simulink model "MPC_backend_adaptive"  (R2026a)
settings: Solver=VariableStepAuto
model workspace (MAT data in the model file):
  kappa_ref = 1
  mpc_ref = 1
undefined symbols (not defined in the file or in its folder): controllerParams
libraries: mpclib x1
settings Model: Creator=rayyu  LastModifiedBy=rayyu
settings DebuggingCC: UnderSpecifiedDimensionMsg=warning

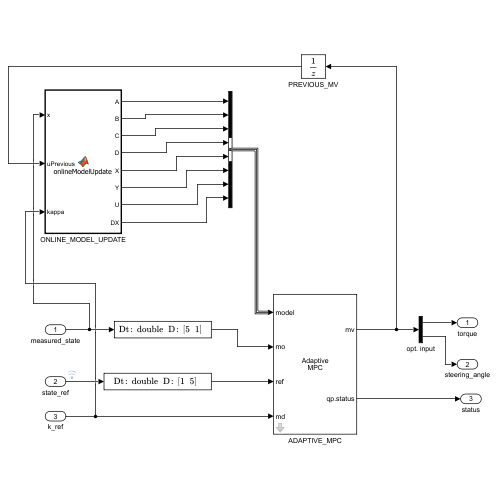
[thumbnail: Simulink's stored preview of the top-level diagram]
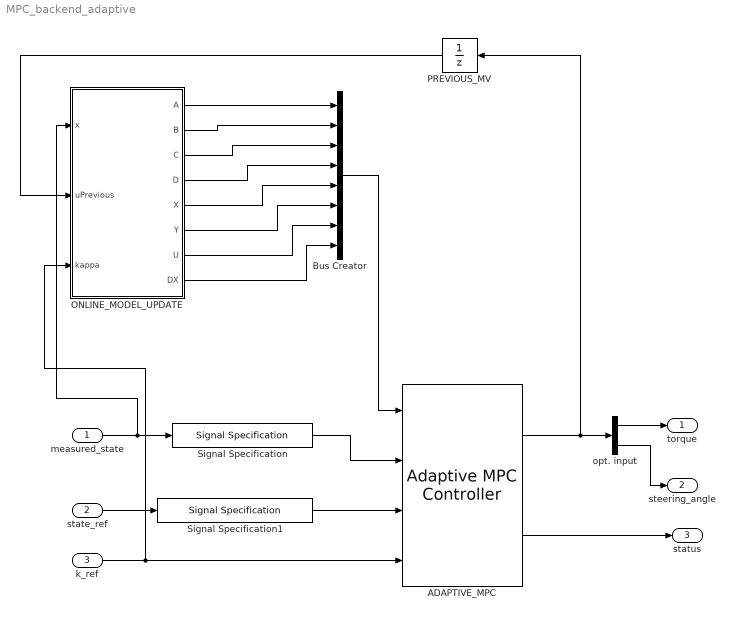
== system MPC_backend_adaptive ==
  measured_state : Inport  PortDimensions=5
  state_ref : Inport  Port=2  PortDimensions=[1 5]
  k_ref : Inport  Port=3
  ADAPTIVE_MPC : mpclib/Adaptive MPC Controller  SCDEnableBlockLinearizationSpecification=on  mpcobj=mpc_adaptive  enable_value=0  updateMPCinCallerWorkspace=on  md_inport=on  mv_inport=off  uref_inport=off  return_cost=off  return_mvseq=off  return_qpstatus=on  return_xseq=off  return_state=off  return_ovseq=off  state_inport=off  isltv_plant=off  umin_inport=off  umax_inport=off  ymin_inport=off  ymax_inport=off  cc_inport=off  ywt_inport=off  uwt_inport=off  duwt_inport=off  rhoeps_inport=off  pm_inport=off  MaximumP=10  HorizonChoice=FixedHorizon  BlockDataType=double  SampleTimeInherited=off  switch_inport=off
  Bus Creator : BusCreator  Inputs=8
  ONLINE_MODEL_UPDATE : MATLAB Function  TreatAsAtomicUnit=on
  PREVIOUS_MV : UnitDelay  InitialCondition=|  SampleTime=controllerParams.Ts_s
      | [
      | controllerParams.nominal_signed_front_axle_torque_Nm
      | controllerParams.nominal_road_wheel_angle_rad
      | ]
  Signal Specification : SignalSpecification  OutDataTypeStr=double  Dimensions=[5 1]
  Signal Specification1 : SignalSpecification  OutDataTypeStr=double  Dimensions=[1 5]
  opt. input : Demux  Outputs=2
  torque : Outport
  steering_angle : Outport  Port=2
  status : Outport  Port=3
  wires:
  ADAPTIVE_MPC/1 -> opt. input/1, PREVIOUS_MV/1
  ADAPTIVE_MPC/2 -> status/1
  measured_state/1 -> ONLINE_MODEL_UPDATE/1(x), Signal Specification/1
  k_ref/1 -> ONLINE_MODEL_UPDATE/3(kappa), ADAPTIVE_MPC/4
  opt. input/1 -> torque/1
  opt. input/2 -> steering_angle/1
  state_ref/1 -> Signal Specification1/1
  Signal Specification/1 -> ADAPTIVE_MPC/2
  Signal Specification1/1 -> ADAPTIVE_MPC/3
  PREVIOUS_MV/1 -> ONLINE_MODEL_UPDATE/2(uPrevious)
  ONLINE_MODEL_UPDATE/1(A) -> Bus Creator/1
  ONLINE_MODEL_UPDATE/2(B) -> Bus Creator/2
  ONLINE_MODEL_UPDATE/3(C) -> Bus Creator/3
  ONLINE_MODEL_UPDATE/4(D) -> Bus Creator/4
  ONLINE_MODEL_UPDATE/5(X) -> Bus Creator/5
  ONLINE_MODEL_UPDATE/6(Y) -> Bus Creator/6
  ONLINE_MODEL_UPDATE/7(U) -> Bus Creator/7
  ONLINE_MODEL_UPDATE/8(DX) -> Bus Creator/8
  Bus Creator/1 -> ADAPTIVE_MPC/1

== matlab function MPC_backend_adaptive/ONLINE_MODEL_UPDATE ==
  data: x input size=[5 1]; A output size=[5 5]; uPrevious input size=[2 1]; kappa input size=[1 1]; B output size=[5 3]; C output size=[5 5]; D output size=[5 3]; X output size=[5 1]; Y output size=[5 1]; U output size=[3 1]; DX output size=[5 1]; adaptiveModelParams parameter
function [A,B,C,D,X,Y,U,DX] = ...
    onlineModelUpdate(x,uPrevious,kappa, adaptiveModelParams)
%#codegen

[A,B,C,D,X,Y,U,DX] = ...
    adaptive_model_update( ...
        x, ...
        uPrevious, ...
        kappa, ...
        adaptiveModelParams);
end
